simulink model "case5"  (Simulink 5.0)
settings: Solver=FixedStepDiscrete  SolverMode=SingleTasking  StartTime=0.0  StopTime=1  FixedStep=Ts  RelTol=1e-3  AbsTol=1e-2
PreLoadFcn:
  | assignin('base','Ts',[50e-6])
undefined symbols (not defined in the file): D1, Delta, Ts
libraries: powerlib2 x68, powerlib_extras x7
settings Model: Creator=sybille  LastModifiedBy=gnedin pa  ExtModeTrigMode=oneshot  ExtModeArmWhenConnect=off  SaveTime=off  LimitDataPoints=off  UnconnectedInputMsg=none  UnconnectedOutputMsg=none  BooleanDataType=off

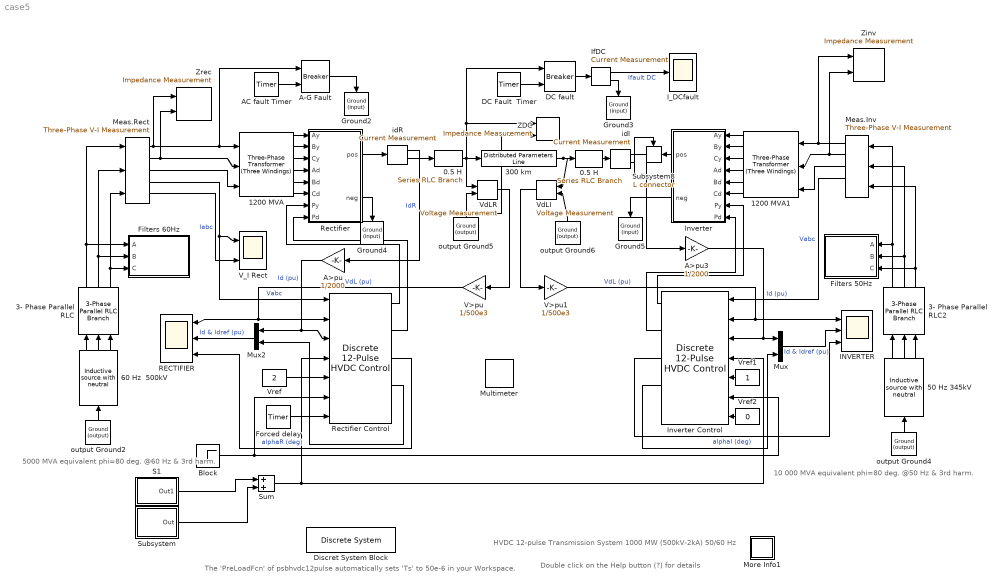
== system case5 ==
  note: 5000 MVA equivalent
      | phi=80 deg. @60 Hz & 3rd harm.
  note: 10 000 MVA equivalent
      | phi=80 deg. @50 Hz & 3rd harm.
  note: The 'PreLoadFcn' of psbhvdc12pulse
      | automatically sets 'Ts' to 50e-6 in your Workspace.
  note: HVDC 12-pulse Transmission System 1000 MW
      |  (500kV-2kA)   50/60 Hz
  note: Double click on the Help button (?) for details
  " 50 Hz 345kV  " : powerlib_extras/Three-Phase Library/Inductive source with neutral  Orientation=up  V=345e3/sqrt(3)*sqrt(2)  Phi=0  F=50  R=0  L=28.0e-3
  " 60 Hz  500kV" : powerlib_extras/Three-Phase Library/Inductive source with neutral  Orientation=up  V=500e3/sqrt(3)*sqrt(2)  Phi=0  F=60  R=0  L=98.03e-3
  0.5 H : powerlib2/Elements/Series RLC Branch  Tag=PoWeRsYsTeMbLoCk  a=1  b=0.5  c=inf  mesure=None  PSBOutputType=1
  "0.5 H " : powerlib2/Elements/Series RLC Branch  Tag=PoWeRsYsTeMbLoCk  a=1  b=0.5  c=inf  mesure=None  PSBOutputType=1
  1200 MVA : powerlib2/Elements/Three-Phase Transformer (Three Windings)  Tag=PoWeRsYsTeMbLoCk  confi=ABC as input terminals  nom=[ 1200e6 , 60 ]  ydw1=Yg  w1="[ 500e3*0.9 0.0025  0 ]"  ydw2=Y  w2=[ 200e3 0.0025 0.24]  ydw3=Delta (D1)  w3=[ 200e3 0.0025 0.24 ]  ynsat=off  rmag=500  lm=500  sat=[0 0; 1 1.2; 2 1.1]  hyst=off  matfile='hysteresis'  sif=off  ifl=[0.8 -0.8 0.7]  initialslopes=[+1 +1 +1]  mesure=None  PSBOutputType=111111
  1200 MVA1 : powerlib2/Elements/Three-Phase Transformer (Three Windings)  Tag=PoWeRsYsTeMbLoCk  Orientation=left  confi=ABC as input terminals  nom=[ 1200e6 , 50 ]  ydw1=Yg  w1="[ 345e3*0.96 0.0025  0 ]"  ydw2=Y  w2="[ 200e3  0.0025 0.24]"  ydw3=Delta (D1)  w3=[ 200e3 0.0025 0.24 ]  ynsat=off  rmag=500  lm=500  sat=[0 0; 1 1.2; 2 1.1]  hyst=off  matfile='hysteresis'  sif=off  ifl=[0.8 -0.8 0.7]  initialslopes=[+1 +1 +1]  mesure=None  PSBOutputType=111111
  3- Phase Parallel RLC : powerlib2/Elements/3-Phase Parallel RLC Branch  Orientation=up  R=26.07  L=48.86e-3  C=0
  3- Phase Parallel RLC2 : powerlib2/Elements/3-Phase Parallel RLC Branch  Orientation=up  R=6.205  L=13.96e-3  C=0
  300 km : powerlib2/Elements/Distributed Parameters Line  Tag=PoWeRsYsTeMbLoCk  n=1  f=60  r=0.015  l=0.792e-3  c=14.4e-9  lgt=300  x1=[0 0 0 0; 0.0001244 0 0 0; 0.0002488 0 0 0; 0.0003733 0 0 0; 0.0004977 0 0 0; 0.0006221 0 0 0]  x2=[0 0 0 0; 0.0001244 0 0 0; 0.0002488 0 0 0; 0.0003733 0 0 0; 0.0004977 0 0 0; 0.0006221 0 0 0]  x3=[0 0 0 0; 0.0001244 0 0 0; 0.0002488 0 0 0; 0.0003733 0 0 0; 0.0004977 0 0 0; 0.0006221 0 0 0]  x4=[0 0 0 0; 0.0001244 0 0 0; 0.0002488 0 0 0; 0.0003733 0 0 0; 0.0004977 0 0 0; 0.0006221 0 0 0]  x5=0  mesure=None  PSBOutputType=111111111111111111111111111111
  A-G Fault : powerlib2/Elements/Breaker  Tag=PoWeRsYsTeMbLoCk  a=0.01  c=0  rs=inf  cs=inf  times="[ 4/60  5/60 ]"  Ts=0  comext=on  mesure=None  PSBOutputType=1
  A>pu : Gain  Orientation=left  Gain=1/2000  SaturateOnIntegerOverflow=on
  A>pu3 : Gain  Gain=1/2000  SaturateOnIntegerOverflow=on
  AC fault Timer : powerlib_extras/Control  Blocks/Timer  t=[ 0.6 0.7]*100  e=[ 1 0 ]
  Block : Step  Time=0.02  Before=1  After=0  SampleTime=0
  DC Fault  Timer : powerlib_extras/Control  Blocks/Timer  t=[0.6 0.65]*100  e=[ 1 0 ]
  DC fault : powerlib2/Elements/Breaker  Tag=PoWeRsYsTeMbLoCk  a=1  c=0  rs=inf  cs=inf  times="[ 4/60  5/60 ]"  Ts=0  comext=on  mesure=None  PSBOutputType=1
  Discret System Block : powerlib2/Discrete System  methode=off  Ts=Ts
  Filters 50Hz : Subsystem  Orientation=left
      mask Display: disp('AC filters\n50 Hz\n600 Mvar')
  Filters 60Hz : Subsystem
      mask Display: disp('AC filters \n60 Hz\n600 Mvar')
  Forced delay : powerlib_extras/Control  Blocks/Timer  t=[0.65 0.7]*100  e=[ 1 0 ]
  Ground{2..5} (4 alike) : powerlib2/Connectors/Ground (input)  Tag=PoWeRsYsTeMbLoCk  Orientation=down
  INVERTER : Scope  NumInputPorts=3
      settings: TimeRange=1  YMin=0.955~1~142.11  YMax=0.99~1.03~142.17  DataFormat=Array  SampleInput=on  SampleTime=Ts
  I_DCfault : Scope
      settings: TimeRange=1  YMin=-1000  YMax=6000  DataFormat=Array  Decimation=Ts  SampleInput=on  SampleTime=Ts
  IfDC : powerlib2/Measurements/Current Measurement  Tag=PoWeRsYsTeMmEaSuReMeNt  PhasorSimulation=off  OutputType=Magnitude  PSBOutputType=01  PSBequivalent=0
  Inverter : Subsystem  Orientation=left
      mask Display: plot(0,0,100,100,[30 70 50 30 ], [60 60 40 60], [50 50], [25 40], [50 50], [ 60 75], [30 70], [40 40], [50 60 70], [40 30 30]);
  Inverter Control : powerlib_extras/Discrete  Control Blocks/Discrete 12-Pulse HVDC Control   Orientation=left  Mode=Inverter  f0Pw=[50 101.5]  XPILimR=[165, 5]  XLinR=[60, 20]  XPILimI=[165, 92]  XLinI="[160,  120]"  Xmarg="[0.1,  0.05]"  XKPI_I=[45, 4500, 90]  XKPI_V="[35, 2250,  90]"  T1_I=0.3e-3  XT_V=[10e-3 , 0.1e-3]  BP=25  Xvdcol=[0.6, 0.18, 0.30, 0.1, 0.080]  alpha_const=off  alpha_fix=165  pas=Ts
  Meas.Inv : powerlib2/Measurements/Three-Phase V-I Measurement  Tag=PoWeRsYsTeMmEaSuReMeNt  Orientation=left  VChoice=phase-to-ground  ualv=off  labelV=V1  Vpu=on  Vbase=345e3  IChoice=yes  ualc=off  labelC=I1  Ppu=on  Pbase=100e6  OutputType=Complex  PhasorSimulation=off  PSBequivalent=0  PSBOutputType=11100
  Meas.Rect : powerlib2/Measurements/Three-Phase V-I Measurement  Tag=PoWeRsYsTeMmEaSuReMeNt  VChoice=phase-to-ground  ualv=off  labelV=V1  Vpu=on  Vbase=500e3  IChoice=yes  ualc=off  labelC=I1  Ppu=on  Pbase=100e6  OutputType=Complex  PhasorSimulation=off  PSBequivalent=0  PSBOutputType=11100
  More Info1 : Subsystem
      mask Display: disp('?')
  Multimeter : powerlib2/Measurements/Multimeter  Tag=PoWeRsYsTeMmEaSuReMeNt  PhasorSimulation=off  OutputType=Magnitude  sel=[1 11 13]  L=16  Gain=[1 1 1]  yselected={'Usw1: Rectifier/Universal Bridge','Isw1: Rectifier/Universal Bridge','Isw3: Rectifier/Universal Bridge'};  PSBOutputType=1  PSBequivalent=0  AxesSetting=[0,0.1,-100,100]  Display=1  SavedBlockNames=-11
  Mux : Mux  Inputs=2
  Mux2 : Mux  Orientation=left  Inputs=2
  RECTIFIER : Scope  NumInputPorts=3
      settings: TimeRange=1  YMin=-0.075~-0.02~89.9  YMax=0.175~0.06~91.2  DataFormat=Array  Decimation=Ts  SampleInput=on  SampleTime=Ts
  Rectifier : Subsystem
      mask Display: plot(0,0,100,100,[30 70 50 30 ], [40 40 60 40], [50 50], [25 40], [50 50], [ 60 75], [30 70], [60 60], [50 40 30], [60 70 70]);
  Rectifier Control : powerlib_extras/Discrete  Control Blocks/Discrete 12-Pulse HVDC Control   Mode=Rectifier  f0Pw=[60 101.5]  XPILimR=[165, 5]  XLinR=[60, 20]  XPILimI=[165, 92]  XLinI="[160,  120]"  Xmarg="[0.1,  0.05]"  XKPI_I=[45, 4500, 90]  XKPI_V=[35, 2250, 90]  T1_I=0.3e-3  XT_V=[10e-3 , 0.1e-3]  BP=30  Xvdcol=[0.6, 0.18, 0.30, 0.1, 0.080]  alpha_const=off  alpha_fix=165  pas=Ts
  S1 : Subsystem  mask(RAMPING UNIT){F_up=1.0, up_slope=1.0/0.4, T_up=0.02, F_down=0., down_slope=-1, T_down=100}
      mask prompts: F_up "Final Up Value (pu):"; up_slope "Up Slope (pu/s):"; T_up "Start Up Time (s):"; F_down "Final Down Value (pu):"; down_slope "Down Slope (pu/s):"; T_down "Start Down Time (s):"
      mask init:
      | T_up_final      =  T_up + F_up/up_slope;
      | T_down_final =   T_down + (F_down-F_up)/down_slope;
      | T_ramp  = [0, T_up, T_up_final,  T_down,  T_down_final, 9999]';
      | U_ramp = [0, 0 , F_up,  F_up,  F_down,  F_down]';
      mask Display: disp('Ramping\n Unit')
  Subsystem : Subsystem
      mask Display: disp('Step Up\n & Down')
  Subsystem8 : powerlib2/Connectors/L connector  Tag=PoWeRsYsTeMbLoCk  Orientation=left
  Sum : Sum  SaturateOnIntegerOverflow=on  InputSameDT=on
  V>pu : Gain  Orientation=left  Gain=1/500e3  SaturateOnIntegerOverflow=on
  V>pu1 : Gain  Gain=1/500e3  SaturateOnIntegerOverflow=on
  V_I Rect : Scope  NumInputPorts=2
      settings: TimeRange=1  YMin=-1.5~-0.75  YMax=1.5~0.75  DataFormat=Array  Decimation=Ts  SampleInput=on  SampleTime=Ts
  VdLI : powerlib2/Measurements/Voltage Measurement  Tag=PoWeRsYsTeMmEaSuReMeNt  Orientation=left  PhasorSimulation=off  OutputType=Magnitude  PSBOutputType=0  PSBequivalent=0
  VdLR : powerlib2/Measurements/Voltage Measurement  Tag=PoWeRsYsTeMmEaSuReMeNt  PhasorSimulation=off  OutputType=Magnitude  PSBOutputType=0  PSBequivalent=0
  Vref : Constant  Value=2
  Vref1 : Constant  Orientation=left
  Vref2 : Constant  Orientation=left  Value=0
  ZDC : powerlib2/Measurements/Impedance Measurement  Tag=PoWeRsYsTeMbLoCk  kz=1
  Zinv : powerlib2/Measurements/Impedance Measurement  Tag=PoWeRsYsTeMbLoCk  kz=0.5
  Zrec : powerlib2/Measurements/Impedance Measurement  Tag=PoWeRsYsTeMbLoCk  kz=0.5
  idI : powerlib2/Measurements/Current Measurement  Tag=PoWeRsYsTeMmEaSuReMeNt  PhasorSimulation=off  OutputType=Magnitude  PSBOutputType=01  PSBequivalent=0
  idR : powerlib2/Measurements/Current Measurement  Tag=PoWeRsYsTeMmEaSuReMeNt  PhasorSimulation=off  OutputType=Magnitude  PSBOutputType=01  PSBequivalent=1
  output Ground{2,4..6} (4 alike) : powerlib2/Connectors/Ground (output)  Tag=PoWeRsYsTeMbLoCk  Orientation=up  PSBOutputType=1
  wires:
  Meas.Rect/2 -> 1200 MVA/2, Zrec/2
  Meas.Rect/3 -> 1200 MVA/3
  idR/2 -> "0.5 H "/1
  idI/2 -> Subsystem8/Enable
  1200 MVA/4 -> Rectifier/4(Ad)
  1200 MVA/6 -> Rectifier/6(Cd)
  1200 MVA/5 -> Rectifier/5(Bd)
  0.5 H/1 -> idI/1
  1200 MVA/1 -> Rectifier/1(Ay)
  1200 MVA/2 -> Rectifier/2(By)
  1200 MVA/3 -> Rectifier/3(Cy)
  DC fault/1 -> IfDC/1
  IfDC/2 -> Ground3/1
  Meas.Rect/1 -> 1200 MVA/1, A-G Fault/1, Zrec/1
  Meas.Rect/5 -> V_I Rect/2  "Iabc"
  output Ground2/1 -> " 60 Hz  500kV"/1
  IfDC/1 -> I_DCfault/1  "Ifault DC"
  A-G Fault/1 -> Ground2/1
  Inverter/2(neg) -> Ground5/1
  Inverter/1(pos) -> Subsystem8/1
  1200 MVA1/1 -> Inverter/1(Ay)
  1200 MVA1/2 -> Inverter/2(By)
  1200 MVA1/3 -> Inverter/3(Cy)
  1200 MVA1/4 -> Inverter/4(Ad)
  1200 MVA1/5 -> Inverter/5(Bd)
  1200 MVA1/6 -> Inverter/6(Cd)
  Meas.Inv/1 -> 1200 MVA1/1, Zinv/1
  Meas.Inv/2 -> 1200 MVA1/2, Zinv/2
  Meas.Inv/3 -> 1200 MVA1/3
  Vref/1 -> Rectifier Control/5
  Rectifier Control/1 -> Rectifier/7(Py)
  Rectifier Control/2 -> Rectifier/8(Pd)
  Rectifier Control/3 -> RECTIFIER/3  "alphaR (deg)"
  Inverter Control/2 -> Inverter/8(Pd)
  Meas.Inv/4 -> Inverter Control/1  "Vabc"
  Inverter Control/1 -> Inverter/7(Py)
  Inverter Control/3 -> INVERTER/3  "alphaI (deg)"
  output Ground4/1 -> " 50 Hz 345kV  "/1
  idR/1 -> A>pu/1  "IdR"
  V>pu/1 -> Rectifier Control/2, RECTIFIER/1  "VdL (pu)"
  Mux/1 -> INVERTER/2  "Id & Idref (pu)"
  idI/1 -> A>pu3/1
  Mux2/1 -> RECTIFIER/2  "Id & Idref (pu)"
  A>pu/1 -> Rectifier Control/3, Mux2/1  "Id (pu)"
  Rectifier Control/4 -> Mux2/2
  "0.5 H "/1 -> VdLR/1, 300 km/1, DC fault/1, ZDC/1
  output Ground5/1 -> VdLR/2, ZDC/2
  VdLR/1 -> V>pu/1
  300 km/1 -> 0.5 H/1, VdLI/1
  output Ground6/1 -> VdLI/2
  VdLI/1 -> V>pu1/1
  V>pu1/1 -> Inverter Control/2, INVERTER/1  "VdL (pu)"
  A>pu3/1 -> Mux/1, Inverter Control/3  "Id (pu)"
  Inverter Control/4 -> Mux/2
  Rectifier/1(pos) -> idR/1
  Rectifier/2(neg) -> Ground4/1
  Vref1/1 -> Inverter Control/5
  Block/1 -> Rectifier Control/6, Inverter Control/6
  AC fault Timer/1 -> A-G Fault/2
  S1/1(Out1) -> Sum/1
  Sum/1 -> Rectifier Control/4, Inverter Control/4
  Vref2/1 -> Inverter Control/7
  DC Fault  Timer/1 -> DC fault/2
  Forced delay/1 -> Rectifier Control/7
  Meas.Rect/4 -> Rectifier Control/1, V_I Rect/1  "Vabc"
  " 60 Hz  500kV"/1 -> 3- Phase Parallel RLC/1
  " 60 Hz  500kV"/2 -> 3- Phase Parallel RLC/2
  " 60 Hz  500kV"/3 -> 3- Phase Parallel RLC/3
  " 50 Hz 345kV  "/1 -> 3- Phase Parallel RLC2/1
  " 50 Hz 345kV  "/2 -> 3- Phase Parallel RLC2/2
  " 50 Hz 345kV  "/3 -> 3- Phase Parallel RLC2/3
  3- Phase Parallel RLC/1 -> Meas.Rect/1, Filters 60Hz/1(A)
  3- Phase Parallel RLC/2 -> Meas.Rect/2, Filters 60Hz/2(B)
  3- Phase Parallel RLC/3 -> Meas.Rect/3, Filters 60Hz/3(C)
  3- Phase Parallel RLC2/1 -> Meas.Inv/1, Filters 50Hz/1(A)
  3- Phase Parallel RLC2/2 -> Meas.Inv/2, Filters 50Hz/2(B)
  3- Phase Parallel RLC2/3 -> Meas.Inv/3, Filters 50Hz/3(C)
  Subsystem/1(Out) -> Sum/2

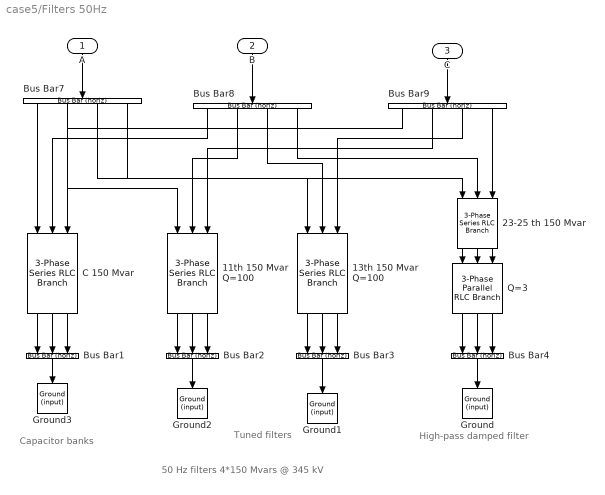
== system case5/Filters 50Hz ==
  note: 50 Hz filters 4*150 Mvars @ 345 kV
  note: Capacitor banks
  note: Tuned filters
  note: High-pass
      | damped filter
  A : Inport  Orientation=down
  B : Inport  Orientation=down  Port=2
  C : Inport  Orientation=down  Port=3
  " 23-25 th 150 Mvar" : powerlib2/Elements/3-Phase Series RLC Branch   Orientation=down  R=0  L=0  C=4.012e-6
  "11th 150 Mvar Q=100 " : powerlib2/Elements/3-Phase Series RLC Branch   Orientation=down  R=0.7214  L=20.87e-3  C=4.012e-6
  13th 150 Mvar Q=100 : powerlib2/Elements/3-Phase Series RLC Branch   Orientation=down  R=0.6104  L=14.95e-3  C=4.012e-6
  Bus Bar{1..4} (4 alike) : powerlib2/Connectors/Bus Bar (horiz)  Tag=PoWeRsYsTeMbLoCk  Orientation=down  entrees=3  sorties=1  PSBOutputType=1111111111111111111111111111111111111111111111111111111111111111111111111
  Bus Bar7 : powerlib2/Connectors/Bus Bar (horiz)  Tag=PoWeRsYsTeMbLoCk  Orientation=down  entrees=1  sorties=4  PSBOutputType=1111111111111111111111111111111111111111111111111111111111111111111111111
  Bus Bar8 : powerlib2/Connectors/Bus Bar (horiz)  Tag=PoWeRsYsTeMbLoCk  Orientation=down  entrees=1  sorties=4  PSBOutputType=1111111111111111111111111111111111111111111111111111111111111111111111111
  Bus Bar9 : powerlib2/Connectors/Bus Bar (horiz)  Tag=PoWeRsYsTeMbLoCk  Orientation=down  entrees=1  sorties=4  PSBOutputType=1111111111111111111111111111111111111111111111111111111111111111111111111
  C 150 Mvar : powerlib2/Elements/3-Phase Series RLC Branch   Orientation=down  R=0  L=0  C=4.012e-6
  Ground{,1..3} (4 alike) : powerlib2/Connectors/Ground (input)  Tag=PoWeRsYsTeMbLoCk  Orientation=down
  Q=3 : powerlib2/Elements/3-Phase Parallel RLC Branch  Orientation=down  R=99.19  L=4.385e-3  C=0
  wires:
  A/1 -> Bus Bar7/1
  B/1 -> Bus Bar8/1
  C/1 -> Bus Bar9/1
  13th 150 Mvar Q=100/1 -> Bus Bar3/1
  13th 150 Mvar Q=100/2 -> Bus Bar3/2
  13th 150 Mvar Q=100/3 -> Bus Bar3/3
  Q=3/1 -> Bus Bar4/1
  Q=3/2 -> Bus Bar4/2
  Q=3/3 -> Bus Bar4/3
  Bus Bar7/1 -> C 150 Mvar/1
  Bus Bar8/1 -> C 150 Mvar/2
  Bus Bar8/3 -> 13th 150 Mvar Q=100/2
  Bus Bar8/4 -> " 23-25 th 150 Mvar"/2
  Bus Bar7/3 -> 13th 150 Mvar Q=100/1
  Bus Bar7/4 -> " 23-25 th 150 Mvar"/1
  Bus Bar9/1 -> C 150 Mvar/3
  Bus Bar9/3 -> 13th 150 Mvar Q=100/3
  Bus Bar9/4 -> " 23-25 th 150 Mvar"/3
  C 150 Mvar/1 -> Bus Bar1/1
  C 150 Mvar/2 -> Bus Bar1/2
  C 150 Mvar/3 -> Bus Bar1/3
  Bus Bar1/1 -> Ground3/1
  "11th 150 Mvar Q=100 "/1 -> Bus Bar2/1
  "11th 150 Mvar Q=100 "/2 -> Bus Bar2/2
  "11th 150 Mvar Q=100 "/3 -> Bus Bar2/3
  Bus Bar8/2 -> "11th 150 Mvar Q=100 "/2
  Bus Bar7/2 -> "11th 150 Mvar Q=100 "/1
  Bus Bar9/2 -> "11th 150 Mvar Q=100 "/3
  Bus Bar2/1 -> Ground2/1
  Bus Bar3/1 -> Ground1/1
  Bus Bar4/1 -> Ground/1
  " 23-25 th 150 Mvar"/1 -> Q=3/1
  " 23-25 th 150 Mvar"/2 -> Q=3/2
  " 23-25 th 150 Mvar"/3 -> Q=3/3

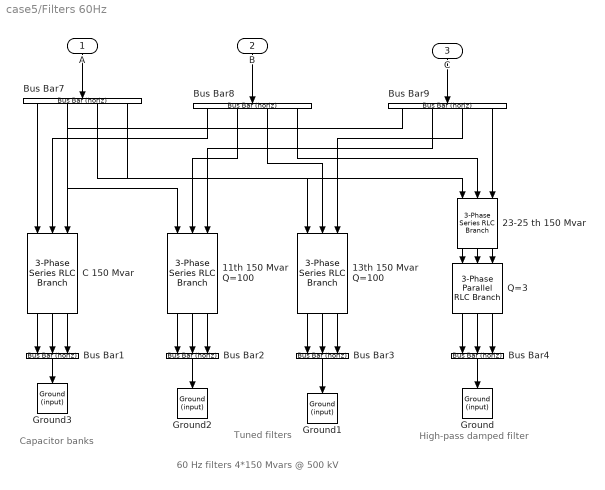
== system case5/Filters 60Hz ==
  note: 60 Hz filters 4*150 Mvars @ 500 kV
  note: High-pass
      | damped filter
  note: Tuned filters
  note: Capacitor banks
  A : Inport  Orientation=down
  B : Inport  Orientation=down  Port=2
  C : Inport  Orientation=down  Port=3
  " 23-25 th 150 Mvar" : powerlib2/Elements/3-Phase Series RLC Branch   Orientation=down  R=0  L=0  C=1.592e-6
  "11th 150 Mvar Q=100 " : powerlib2/Elements/3-Phase Series RLC Branch   Orientation=down  R=1.515  L=36.53e-3  C=1.592e-6
  13th 150 Mvar Q=100 : powerlib2/Elements/3-Phase Series RLC Branch   Orientation=down  R=1.282  L=26.15e-3  C=1.592e-6
  Bus Bar{1..4} (4 alike) : powerlib2/Connectors/Bus Bar (horiz)  Tag=PoWeRsYsTeMbLoCk  Orientation=down  entrees=3  sorties=1  PSBOutputType=1111111111111111111111111111111111111111111111111111111111111111111111111
  Bus Bar7 : powerlib2/Connectors/Bus Bar (horiz)  Tag=PoWeRsYsTeMbLoCk  Orientation=down  entrees=1  sorties=4  PSBOutputType=1111111111111111111111111111111111111111111111111111111111111111111111111
  Bus Bar8 : powerlib2/Connectors/Bus Bar (horiz)  Tag=PoWeRsYsTeMbLoCk  Orientation=down  entrees=1  sorties=4  PSBOutputType=1111111111111111111111111111111111111111111111111111111111111111111111111
  Bus Bar9 : powerlib2/Connectors/Bus Bar (horiz)  Tag=PoWeRsYsTeMbLoCk  Orientation=down  entrees=1  sorties=4  PSBOutputType=1111111111111111111111111111111111111111111111111111111111111111111111111
  C 150 Mvar : powerlib2/Elements/3-Phase Series RLC Branch   Orientation=down  R=0  L=0  C=1.592e-6
  Ground{,1..3} (4 alike) : powerlib2/Connectors/Ground (input)  Tag=PoWeRsYsTeMbLoCk  Orientation=down
  Q=3 : powerlib2/Elements/3-Phase Parallel RLC Branch  Orientation=down  R=208.3  L=7.673e-3  C=0
  wires:
  " 23-25 th 150 Mvar"/3 -> Q=3/3
  " 23-25 th 150 Mvar"/2 -> Q=3/2
  " 23-25 th 150 Mvar"/1 -> Q=3/1
  Bus Bar4/1 -> Ground/1
  Bus Bar3/1 -> Ground1/1
  Bus Bar2/1 -> Ground2/1
  Bus Bar9/2 -> "11th 150 Mvar Q=100 "/3
  Bus Bar7/2 -> "11th 150 Mvar Q=100 "/1
  Bus Bar8/2 -> "11th 150 Mvar Q=100 "/2
  "11th 150 Mvar Q=100 "/3 -> Bus Bar2/3
  "11th 150 Mvar Q=100 "/2 -> Bus Bar2/2
  "11th 150 Mvar Q=100 "/1 -> Bus Bar2/1
  Bus Bar1/1 -> Ground3/1
  C 150 Mvar/3 -> Bus Bar1/3
  C 150 Mvar/2 -> Bus Bar1/2
  C 150 Mvar/1 -> Bus Bar1/1
  Bus Bar9/4 -> " 23-25 th 150 Mvar"/3
  Bus Bar9/3 -> 13th 150 Mvar Q=100/3
  Bus Bar9/1 -> C 150 Mvar/3
  Bus Bar7/4 -> " 23-25 th 150 Mvar"/1
  Bus Bar7/3 -> 13th 150 Mvar Q=100/1
  Bus Bar8/4 -> " 23-25 th 150 Mvar"/2
  Bus Bar8/3 -> 13th 150 Mvar Q=100/2
  Bus Bar8/1 -> C 150 Mvar/2
  Bus Bar7/1 -> C 150 Mvar/1
  Q=3/3 -> Bus Bar4/3
  Q=3/2 -> Bus Bar4/2
  Q=3/1 -> Bus Bar4/1
  13th 150 Mvar Q=100/3 -> Bus Bar3/3
  13th 150 Mvar Q=100/2 -> Bus Bar3/2
  13th 150 Mvar Q=100/1 -> Bus Bar3/1
  C/1 -> Bus Bar9/1
  B/1 -> Bus Bar8/1
  A/1 -> Bus Bar7/1

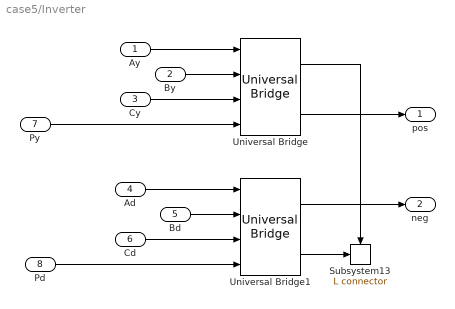
== system case5/Inverter ==
  Ay : Inport
  By : Inport  Port=2
  Cy : Inport  Port=3
  Ad : Inport  Port=4
  Bd : Inport  Port=5
  Cd : Inport  Port=6
  Py : Inport  Port=7
  Pd : Inport  Port=8
  Subsystem13 : powerlib2/Connectors/L connector  Tag=PoWeRsYsTeMbLoCk
  Universal Bridge : powerlib2/Power Electronics/Universal Bridge  Tag=PoWeRsYsTeMbLoCk  arms=3  confi=ABC as input terminals  injcc=2000  cf=0.1e-6  device=Thyristors  Ron=1e-3  Lon=0  VFs="[  0.8  0.8  ]"  Vf=0  gtoparameters=[ 10e-6 , 20e-6 ]  igbtparameters=[ 1e-6 , 2e-6 ]  mesure=None  PSBOutputType=111
  Universal Bridge1 : powerlib2/Power Electronics/Universal Bridge  Tag=PoWeRsYsTeMbLoCk  arms=3  confi=ABC as input terminals  injcc=2000  cf=0.1e-6  device=Thyristors  Ron=1e-3  Lon=0  VFs="[  0.8  0.8  ]"  Vf=0  gtoparameters=[ 10e-6 , 20e-6 ]  igbtparameters=[ 1e-6 , 2e-6 ]  mesure=None  PSBOutputType=111
  pos : Outport
  neg : Outport  Port=2
  wires:
  Pd/1 -> Universal Bridge1/4
  Py/1 -> Universal Bridge/4
  Cd/1 -> Universal Bridge1/3
  Bd/1 -> Universal Bridge1/2
  Ad/1 -> Universal Bridge1/1
  Cy/1 -> Universal Bridge/3
  By/1 -> Universal Bridge/2
  Ay/1 -> Universal Bridge/1
  Universal Bridge/1 -> Subsystem13/Enable
  Universal Bridge1/2 -> Subsystem13/1
  Universal Bridge/2 -> pos/1
  Universal Bridge1/1 -> neg/1

== system case5/More Info1 ==
  note: Notice the 120 Hz oscillations in the DC voltage and currents during the fault. When the fault is cleared at t=0.7 s,
      | the VDCOL operates and reduces the reference current to 0.3 pu. The system recovers in approximately 0.4 s after fault clearing.
  note: In the DC Fault Timer and Forced Delay Timer blocks, change the multiplication factor of 1 in the Transition Times to 100,
      | so that the DC fault is now eliminated.  In the AC Fault timer, change the multiplication factor in the Transition Times to 1,
      | so that a 6 cycles line-to-ground fault is now applied at the rectifier. Restart the simulation.
  note: AC line-to-ground fault
  note: Disconnect the Step Up & Down block in order to eliminate the step disturbance applied on the reference current.
      | In the DC Fault Timer and Forced Delay Timer blocks, change the multiplication factor of 100 in the Transition Times to 1,
      | so that a fault is now applied at t=0.6s. Open the I_DCfault scope to observe the fault current. Restart the simulation.
  note: At fault application the DC current quickly increases to 2.3 pu and the DC voltage falls to zero at the rectifier.
      | This DC voltages drop is seen by the Voltage Dependant Currrent Order Limiter (VDCOL) which reduces the reference current to 0.3 pu at the rectifier.
      | A DC current still continues to circulate in the fault. Then, a t=0.65 s, the rectifier alpha firing angle is forced to 165 degrees by the protection systems (not simulated).
      | The rectifier now operates in inverter mode. The DC line voltage becomes negative and the energy stored in the line is returned to the AC network,
      | causing rapid extinction of the fault current at its next zero-crossing. Then, alpha is released at t=0.7 s and the normal DC voltage and current
      |  recover in approcxximately 0.3 s.
  note: DC line fault
  note: Start-up
  note: DEMONSTRATION
  note: A 1000 MW (500 kV, 2kA) DC linterconnexion is used to transmit power from a 500 kV, 5000 MVA,60Hz network.
      | to a  345 kV, 10 000MVA, 50Hz network.
      |
      | The rectifier and the inverter  are 12-pulse converters using  two 6-pulse Universal briges connected in series.
      | Open the two converter subsystems to see how they are built. The converters are interconnected through a 300 km distributed parameter
      | line through and 0.5 H smoothing reactors. The converter transformers are modelled with Universal Transformer blocks.
      | The transformer tap changers are kept at a fixed tap. Open the two transformer blocks to see the factors applied
      | on the primary voltage (0.90 on rectifier side; 0.96 on inverter side). The reactive power required by the converters is provided
      | by a set of filters (C bank plus 11th, 13th and  high pass filters; total 600 Mvar on each side).
      | Open the AC filter subsystems to see the filter toplogy.  Two circuit breakers are used to apply faults on the rectifier AC and DC sides.
      |
      | The rectifier and inverter control systems use the  Discrete 12-pulse HVDC Control block of the Extras/Control library.
      |  The power system and the control system are both  discretized (Sample time= Ts).
      | A description of the control systems is provided in the HVDC Transmission System Case Study of the User's Manual.
  note: This demonstration  illustrates steady-state and transient performance
      | of a 12-pulse,  1000 MW (500 kV-2kA) 50/60 Hz HVDC transmission system
  note: CIRCUIT DESCRIPTION
  note: Notice that the system is discretized, using sample time Ts; Specify Ts=50e-6 in your Matlab window.
      | The system is programmed to start and  reach a steady state.
      | Then, a step is applied on the reference current to observe the dynamic response of the regulators.
      | Start the simulation and observe the following events on the RECTIFIER and  INVERTER scopes
  note: The reference current is ramped from zero to 1 pu (2kA) in 0.4 s. The DC current and voltages start from zero and reach steady-state
      |  in approximately 0.5 s.The rectifier controls the current and the inverter controls the voltage.Trace 1 of both RECTIFIER and INVERTER scopes
      |  shows the DC line voltage (1pu=500 kV). Trace 2 shows the the reference current and the measured Id current (1pu=2kA).
      | In steady-state, the alpha firing angles (trace 3) are 18 degres and 142 degrees respectively on the rectifier and inverter side.
  note: At t=0.6 s, a 0.2 pu step is applied on the reference current (decrease from 1 pu  to 0.8 pu ).
      | At t=0.75s,another step is applied to set the reference back to 1 pu.
      | Observe the response of the current regulator . It stabilizes in  approximately 0.05 s
  note: Step reponse of regulators
  note: S. Casoria ; Hydro-Quebec (IREQ)

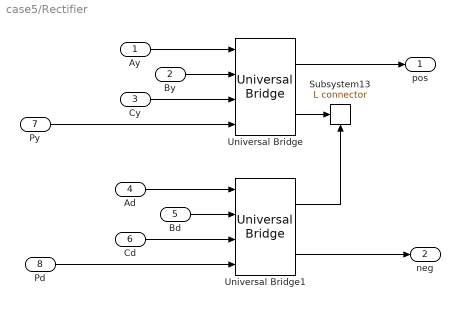
== system case5/Rectifier ==
  Ay : Inport
  By : Inport  Port=2
  Cy : Inport  Port=3
  Ad : Inport  Port=4
  Bd : Inport  Port=5
  Cd : Inport  Port=6
  Py : Inport  Port=7
  Pd : Inport  Port=8
  Subsystem13 : powerlib2/Connectors/L connector  Tag=PoWeRsYsTeMbLoCk  Orientation=up
  Universal Bridge : powerlib2/Power Electronics/Universal Bridge  Tag=PoWeRsYsTeMbLoCk  arms=3  confi=ABC as input terminals  injcc=2000  cf=0.1e-6  device=Thyristors  Ron=1e-3  Lon=0  VFs="[  0.8  0.8  ]"  Vf=0  gtoparameters=[ 10e-6 , 20e-6 ]  igbtparameters=[ 1e-6 , 2e-6 ]  mesure=All voltages and currents  PSBOutputType=111
  Universal Bridge1 : powerlib2/Power Electronics/Universal Bridge  Tag=PoWeRsYsTeMbLoCk  arms=3  confi=ABC as input terminals  injcc=2000  cf=0.1e-6  device=Thyristors  Ron=1e-3  Lon=0  VFs="[  0.8  0.8  ]"  Vf=0  gtoparameters=[ 10e-6 , 20e-6 ]  igbtparameters=[ 1e-6 , 2e-6 ]  mesure=None  PSBOutputType=111
  pos : Outport
  neg : Outport  Port=2
  wires:
  Universal Bridge/2 -> Subsystem13/Enable
  Ay/1 -> Universal Bridge/1
  Universal Bridge/1 -> pos/1
  By/1 -> Universal Bridge/2
  Cy/1 -> Universal Bridge/3
  Ad/1 -> Universal Bridge1/1
  Bd/1 -> Universal Bridge1/2
  Cd/1 -> Universal Bridge1/3
  Universal Bridge1/1 -> Subsystem13/1
  Universal Bridge1/2 -> neg/1
  Py/1 -> Universal Bridge/4
  Pd/1 -> Universal Bridge1/4

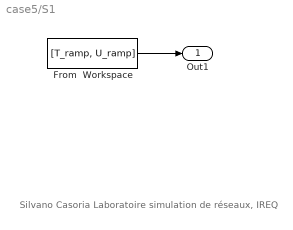
== system case5/S1 ==
  note: Silvano Casoria
      | Laboratoire simulation de réseaux, IREQ
  From  Workspace : FromWorkspace  VariableName="[T_ramp,  U_ramp]"  SampleTime=0
  Out1 : Outport  InitialOutput=0
  wires:
  From  Workspace/1 -> Out1/1

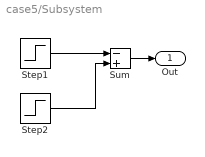
== system case5/Subsystem ==
  Step1 : Step  Time=0.6  After=0.2  SampleTime=0
  Step2 : Step  Time=0.75  After=0.2  SampleTime=0
  Sum : Sum  Inputs=-+  SaturateOnIntegerOverflow=on  InputSameDT=on
  Out : Outport
  wires:
  Step1/1 -> Sum/1
  Step2/1 -> Sum/2
  Sum/1 -> Out/1
